simulink model "FDC2214EVM_rts"  (R2018a)
settings: Solver=FixedStepAuto  StartTime=0.0  StopTime=inf  FixedStep=0.1  RelTol=1e-3  EnableMultiTasking=on
undefined symbols (not defined in the file or in its folder): serial
libraries: instrumentlib x3, xpcseriallib x1, slrtlib x1
settings Model: SimulationMode=external  Creator=aillar  LastModifiedBy=aillar
settings SolverCC: ConcurrentTasks=on  AutoInsertRateTranBlk=on
settings DataIOCC: LimitDataPoints=on  MaxDataPoints=10000  SaveFormat=StructureWithTime  SaveOutput=off  SaveTime=off
settings OptimizationCC: BlockReduction=off  DefaultParameterBehavior=Inlined  UseDivisionForNetSlopeComputation=on  UseFloatMulNetSlope=on  OptimizeBlockIOStorage=off  BufferReuse=off  GlobalBufferReuse=off  ExpressionFolding=off  PassReuseOutputArgsThreshold=0  LocalBlockOutputs=off  EfficientFloat2IntCast=on  OptimizeDataStoreBuffers=off  BusAssignmentInplaceUpdate=off
settings DebuggingCC: AlgebraicLoopMsg=error  SingleTaskRateTransMsg=error  ParameterTunabilityLossMsg=error  AllowSymbolicDim=off  SFUnexpectedBacktrackingDiag=warning  SFNoUnconditionalDefaultTransitionDiag=warning  SFExecutionAtInitializationDiag=none
settings HardwareCC: ProdBitPerPointer=32  ProdBitPerSizeT=32  ProdBitPerPtrDiffT=32  ProdLargestAtomicFloat=None  ProdWordSize=32  ProdLongLongMode=on  ProdHWDeviceType=Generic->32-bit x86 compatible
settings SFSimCC: MATLABDynamicMemAlloc=off
settings RTWCC: SystemTargetFile=slrt.tlc  TemplateMakefile=slrt_default_tmf  Description=Simulink Real-Time  GenerateReport=on  LaunchReport=on  CodeExecutionProfiling=on  RTWCompilerOptimization=on
settings CodeAppCC: ForceParamTrailComments=on  OperatorAnnotations=on
settings SimulinkRealTimeCC: SupportVariableSizeSignals=on  RL32LogTETModifier=off  xPCConcurrentTasks=on
settings ConfigComp: CovMetricSettings=dw  CovHtmlReporting=on  CovSaveCumulativeToWorkspaceVar=on  CovSaveSingleToWorkspaceVar=on  CovExternalEMLEnable=off  CovSFcnEnable=off

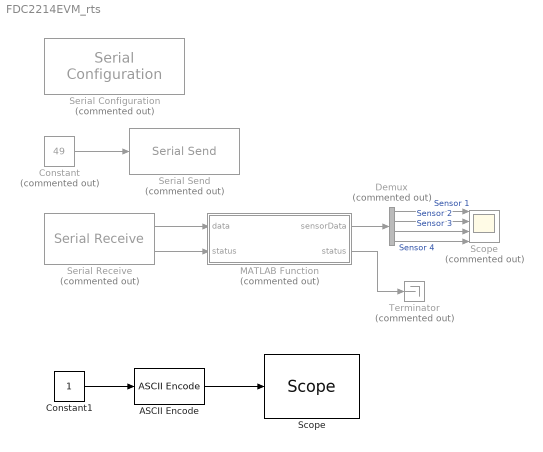
== system FDC2214EVM_rts ==
  "ASCII Encode " : xpcseriallib/ASCII Encode   format=%d\r  nvars=1  maxlength=1  vartypes={ 'uint8' }
      settings: SourceProductName=Simulink Real-Time  SourceProductBaseCode=XP
  Constant : Constant  Commented=on  Value=49  OutDataTypeStr=uint8
  Constant1 : Constant  OutDataTypeStr=uint8
  Demux : Demux  Commented=on
  MATLAB Function : MATLAB Function  Commented=on  TreatAsAtomicUnit=on
  Scope : Scope  Commented=on  NumInputPorts=4
  "Scope " : slrtlib/Displays and Logging/Scope   scopeno=1  scopetype=Target  autostart=on  viewmode=Numerical  formatstr='%15.6f'  grid=on  ylimits=[0,0]  nosamples=3  noprepostsamples=0  interleave=1  triggermode=FreeRun  triggersignal=1  trigsignalfromport=off  triggerlevel=0.0  triggerslope=Either  triggerscope=1  triggersample=0  filename=data.dat  mode=Lazy  writesize=512  autorestart=off  dynamicfilemode=off  maxwritefilesize=512*1024^2
  Serial Configuration : instrumentlib/Serial Configuration  Priority=-200000  Commented=on  ComPortMenu=COM5  ComPort=COM5  ObjConstructor=serial('COM5');  BaudRate=115200  DataBits=8  Parity=none  StopBits=1  FlowControl=none  Timeout=1  ByteOrder=LittleEndian
  Serial Receive : instrumentlib/Serial Receive  Commented=on  ComPortMenu=COM5  ComPort=COM5  ObjConstructor=serial('COM5');  Terminator=<none>  DataSize="[1  37]"  DataType=uint8  EnableBlockingMode=off  ActionDataUnavailable=Output last received value  CustomValue=0  SampleTime=0.001
  Serial Send : instrumentlib/Serial Send  Commented=on  ComPortMenu=COM5  ComPort=COM5  ObjConstructor=serial('COM5');  Terminator=<none>  EnableBlockingMode=off
  Terminator : Terminator  Commented=on
  wires:
  Constant/1 -> Serial Send/1
  Serial Receive/1 -> MATLAB Function/1(data)
  MATLAB Function/1(sensorData) -> Demux/1
  MATLAB Function/2(status) -> Terminator/1
  Demux/1 -> Scope/1  "Sensor 1"
  Demux/2 -> Scope/2  "Sensor 2"
  Demux/3 -> Scope/3  "Sensor 3"
  Demux/4 -> Scope/4  "Sensor 4"
  Serial Receive/2 -> MATLAB Function/2("status ")
  Constant1/1 -> "ASCII Encode "/1
  "ASCII Encode "/1 -> "Scope "/1

== matlab function FDC2214EVM_rts/MATLAB Function ==
  data data settings: description=The Data port contains the set of data from Serial Receive block at each time step.
  data sensorData settings: description=The sensorData containes total (or sensor) capacitance data (in pF) from FDC2214EVM.
  data status settings: description=The Status port contains 0 or 1 based on whether it received new data at the given time step.
  data status settings: description=The Status port contains 0 or 1 based on whether it received new data at the given time step.
  data: data input uint8; sensorData output double size=[1 4]; status input double size=1; status output
function [sensorData, status] = sensorData(data, status)
  parallelInductance  = 18; % 18 muH
  parallelCapacitance = 33; % surface mount capacitance = 33 pF (total capacitance = 53pF)
  fCLK = 40;                % (external) frequency measurement master clock
  
  % Reference clock divider settings
  CH_FREF_DIVIDER = [1, 1, 1, 1];
  CH_FIN_SEL      = [1, 1, 1, 1];
  
  sensorData = zeros(1,4);
  
  if sum(data) ~= 0
    chData = char(data(1:end-2));
    
    sensorData(1,1) = hex2dec(chData(1:8));
    sensorData(1,2) = hex2dec(chData(10:17));
    sensorData(1,3) = hex2dec(chData(19:26));
    sensorData(1,4) = hex2dec(chData(28:35));
    
    % Frequency[MHz], Capacitance[pF]
    frequency = CH_FIN_SEL./CH_FREF_DIVIDER * fCLK/2^28 .* sensorData;
    totalCapacitance = 1./(2*pi*frequency).^2/parallelInductance * 10^6; % fSENSOR = 1/(2*pi*sqrt(LC))
    sensorCapacitance = totalCapacitance - parallelCapacitance;
    
    sensorData = totalCapacitance;
  end
end
